simulink model "QuadCopterSimulation_CL_Original"  (R2024a)
settings: Solver=ode23t  StartTime=0  StopTime=25  RelTol=1e-6  AbsTol=1e-6
values from neighbouring files (symbols this model uses):
  Cd = 5.804e-9    (= 5.804e-09)    [parameters.m]
  Ct = 4.980e-8    (= 4.98e-08)    [parameters.m]
  d = 0.21    [parameters.m]
  g = 9.81    [parameters.m]
  Ixx = 1.467e-2    (= 0.01467)    [parameters.m]
  Iyy = 1.667e-2    (= 0.01667)    [parameters.m]
  Izz = 1.325e-2    (= 0.01325)    [parameters.m]
  m = 0.9    [parameters.m]
libraries: vrlib x9, slpidlib x4
settings Model: SimulationMode=accelerator  SnapshotInterval=1  PacingRate=1.300000  Creator=abdma  LastModifiedBy=abdma
settings SolverCC: AlgebraicLoopSolver=TrustRegion
settings DebuggingCC: UnconnectedInputMsg=warning  UnconnectedOutputMsg=warning  UnconnectedLineMsg=warning  ArithmeticOperatorsInVariantConditions=warning
settings ModelReferenceCC: EnableRefExpFcnMdlSchedulingChecks=on
settings SFSimCC: CustomCodeUndefinedFunction=UseInterfaceOnly
settings RTWCC: GPUComputeCapability=3.5

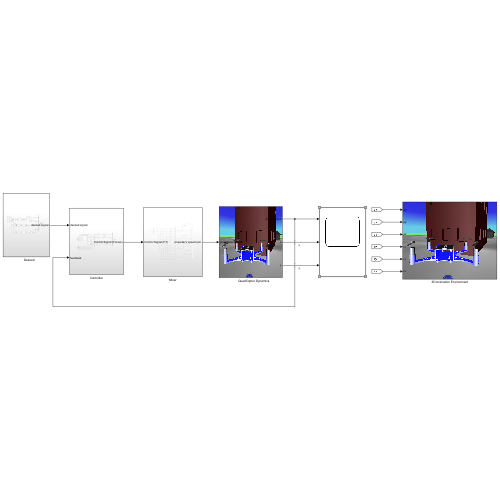
[thumbnail: Simulink's stored preview of the top-level diagram]
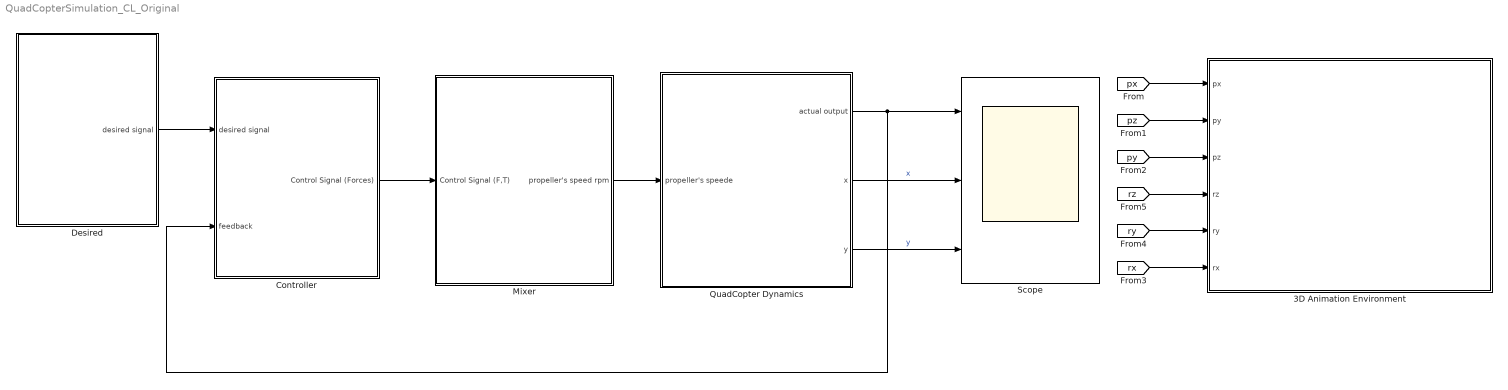
== system QuadCopterSimulation_CL_Original ==
  "\tDesired" : Subsystem
  "\tQuadCopter Dynamics" : Subsystem
      mask Display: image('Capture.PNG');
  3D Animation Environment : Subsystem
      mask Display: image('Capture.PNG');
  Controller : Subsystem
  Mixer : Subsystem
  Scope : Scope  NumInputPorts=3
  wires:
  "\tDesired"/1(desired signal) -> Controller/1(desired signal)
  Controller/1(Control Signal (Forces)) -> Mixer/1(Control Signal (F,T))
  "\tQuadCopter Dynamics"/1(actual output) -> Scope/1, Controller/2(feedback)
  Mixer/1(propeller's speed rpm) -> "\tQuadCopter Dynamics"/1(propeller's speede)
  "\tQuadCopter Dynamics"/2(x) -> Scope/2  "x"
  "\tQuadCopter Dynamics"/3(y) -> Scope/3  "y"
  [px] -> 3D Animation Environment/1(px)
  [pz] -> 3D Animation Environment/2(py)
  [py] -> 3D Animation Environment/3(pz)
  [rz] -> 3D Animation Environment/4(rz)
  [ry] -> 3D Animation Environment/5(ry)
  [rx] -> 3D Animation Environment/6(rx)

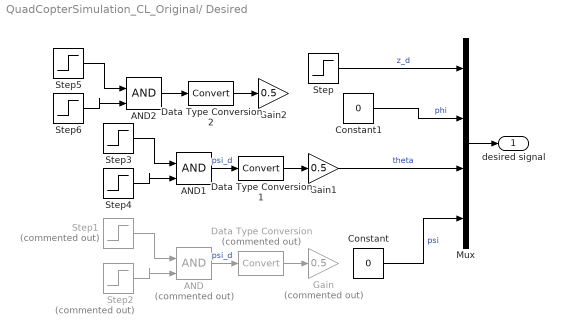
== system QuadCopterSimulation_CL_Original/	Desired ==
  AND : Logic  Commented=on  IconShape=distinctive  AllPortsSameDT=off  OutDataTypeStr=boolean
  AND1 : Logic  IconShape=distinctive  AllPortsSameDT=off  OutDataTypeStr=boolean
  AND2 : Logic  IconShape=distinctive  AllPortsSameDT=off  OutDataTypeStr=boolean
  Constant : Constant  Value=0
  Constant1 : Constant  Value=0
  Data Type Conversion : DataTypeConversion  Commented=on  SaturateOnIntegerOverflow=off  RndMeth=Floor
  Data Type Conversion1 : DataTypeConversion  SaturateOnIntegerOverflow=off  RndMeth=Floor
  Data Type Conversion2 : DataTypeConversion  SaturateOnIntegerOverflow=off  RndMeth=Floor
  Gain : Gain  Commented=on  Gain=0.5
  Gain1 : Gain  Gain=0.5
  Gain2 : Gain  Gain=0.5
  Mux : Mux
  Step : Step  Time=0  After=-5  SampleTime=0
  Step1 : Step  Commented=on  Time=4  SampleTime=0
  Step2 : Step  Commented=on  Time=8  Before=1  After=0  SampleTime=0
  Step3 : Step  Time=8  SampleTime=0
  Step4 : Step  Time=9  Before=1  After=0  SampleTime=0
  Step5 : Step  Time=10  SampleTime=0
  Step6 : Step  Time=11  Before=1  After=0  SampleTime=0
  desired signal : Outport
  wires:
  Step/1 -> Mux/1  "z_d"
  AND/1 -> Data Type Conversion/1  "psi_d"
  Mux/1 -> desired signal/1
  Step1/1 -> AND/1
  Step2/1 -> AND/2
  Data Type Conversion/1 -> Gain/1
  Data Type Conversion1/1 -> Gain1/1
  Step4/1 -> AND1/2
  Step3/1 -> AND1/1
  AND1/1 -> Data Type Conversion1/1  "psi_d"
  Constant/1 -> Mux/4  "psi"
  Gain1/1 -> Mux/3  "theta"
  AND2/1 -> Data Type Conversion2/1
  Step5/1 -> AND2/1
  Step6/1 -> AND2/2
  Data Type Conversion2/1 -> Gain2/1
  Constant1/1 -> Mux/2  "phi"

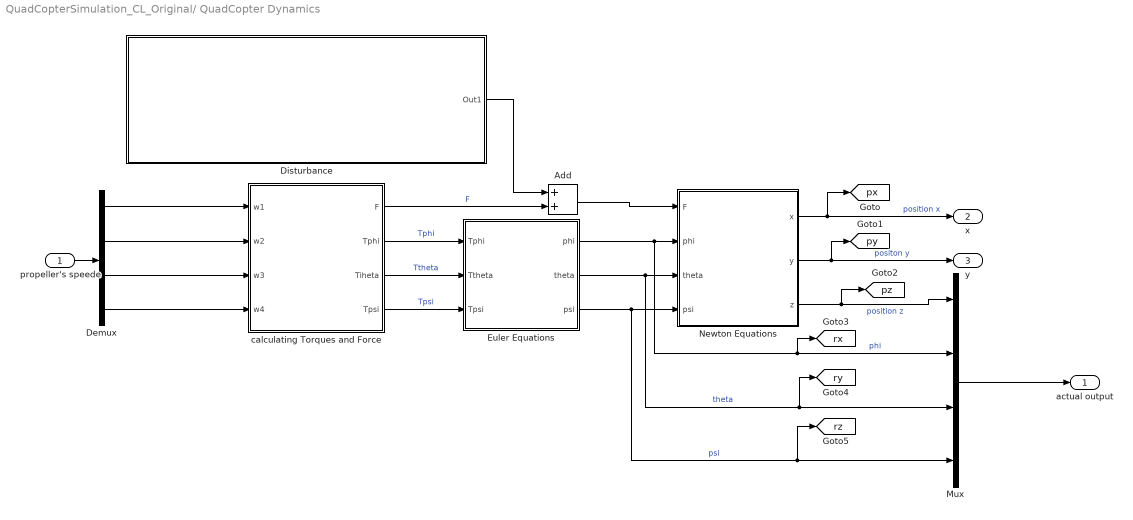
== system QuadCopterSimulation_CL_Original/	QuadCopter Dynamics ==
  propeller's speede : Inport
  Add : Sum
  Demux : Demux
  Disturbance : Subsystem
  Euler Equations : Subsystem
  Mux : Mux
  Newton Equations : Subsystem
  calculating Torques and Force : Subsystem
  actual output : Outport
  x : Outport  Port=2
  y : Outport  Port=3
  tag scope: px=global, py=global, pz=global, rx=global, ry=global, rz=global
  wires:
  Euler Equations/1(phi) -> [rx], Mux/2, Newton Equations/2(phi)  "phi"
  Euler Equations/3(psi) -> [rz], Mux/4, Newton Equations/4(psi)  "psi"
  calculating Torques and Force/3(Tiheta) -> Euler Equations/2(Ttheta)  "Ttheta"
  Euler Equations/2(theta) -> [ry], Mux/3, Newton Equations/3(theta)  "theta"
  calculating Torques and Force/2(Tphi) -> Euler Equations/1(Tphi)  "Tphi"
  Newton Equations/1(x) -> [px], x/1  "position x"
  calculating Torques and Force/4(Tpsi) -> Euler Equations/3(Tpsi)  "Tpsi"
  Newton Equations/2(y) -> [py], y/1  "positon y"
  Newton Equations/3(z) -> [pz], Mux/1  "position z"
  Mux/1 -> actual output/1
  propeller's speede/1 -> Demux/1
  Demux/1 -> calculating Torques and Force/1(w1)
  Demux/2 -> calculating Torques and Force/2(w2)
  Demux/3 -> calculating Torques and Force/3(w3)
  Demux/4 -> calculating Torques and Force/4(w4)
  calculating Torques and Force/1(F) -> Add/2  "F"
  Add/1 -> Newton Equations/1(F)
  Disturbance/1(Out1) -> Add/1

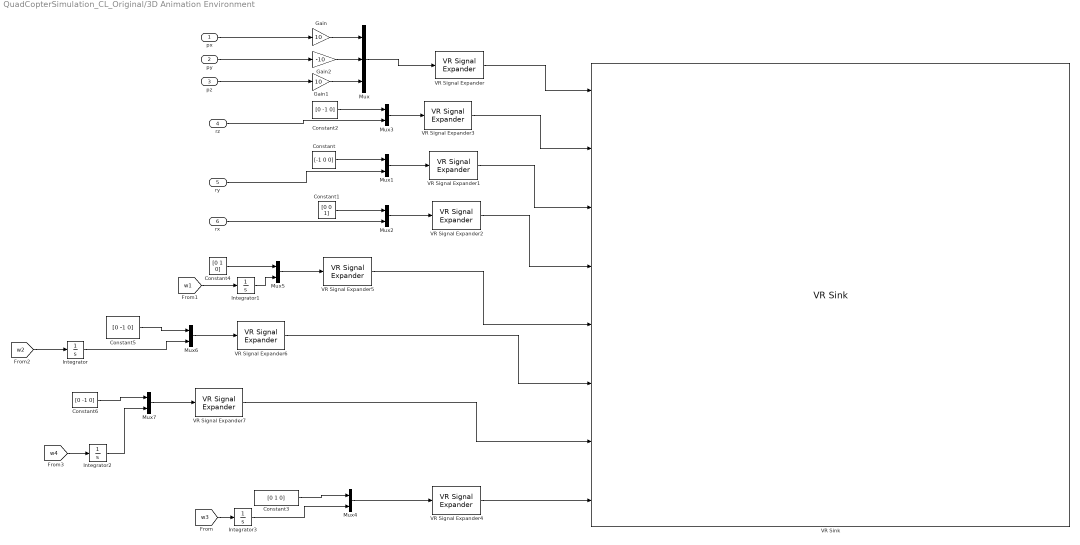
== system QuadCopterSimulation_CL_Original/3D Animation Environment ==
  px : Inport
  py : Inport  Port=2
  pz : Inport  Port=3
  rz : Inport  Port=4
  ry : Inport  Port=5
  rx : Inport  Port=6
  Constant : Constant  Value=[-1 0 0]
  Constant1 : Constant  Value=[0 0 1]
  Constant2 : Constant  Value=[0 -1 0]
  Constant3 : Constant  Value=[0 1 0]
  Constant4 : Constant  Value=[0 1 0]
  Constant5 : Constant  Value=[0 -1 0]
  Constant6 : Constant  Value=[0 -1 0]
  Gain : Gain  Gain=10
  Gain1 : Gain  Gain=10
  Gain2 : Gain  Gain=-10
  Integrator{,1..3} (4 alike) : Integrator
  Mux : Mux  Inputs=3
  Mux{1..7} (7 alike) : Mux  Inputs=2
  VR Signal Expander : vrlib/VR Signal Expander  outwidth=3  outidx=[1 2 3 ]
  VR Signal Expander{1..7} (7 alike) : vrlib/VR Signal Expander  outwidth=4  outidx=[1 2 3 4]
  VR Sink : vrlib/VR Sink  InstantiateOnLoad=on  SampleTime=0.1  ViewEnable=on  RemoteChange=off  RemoteView=off  FieldsWritten=DroneFrame.translation.3.1.1.double#frameZ.rotation.4.1.1.double#frameY.rotation.4.1.1.double#frameX.rotation.4.1.1.double#propeller1.rotation.4.1.1.double#propeller2.rotation.4.1.1.double#propeller4.rotation.4.1.1.double#propeller3.rotation.4.1.1.double  WorldFileName=minidroneassembly.wrl  AutoView=on  VideoDimensions=[]  AllowVariableSize=off
  wires:
  Mux/1 -> VR Signal Expander/1
  Mux3/1 -> VR Signal Expander3/1
  Gain2/1 -> Mux/2
  Gain1/1 -> Mux/3
  rx/1 -> Mux2/2
  Mux1/1 -> VR Signal Expander1/1
  Gain/1 -> Mux/1
  rz/1 -> Mux3/2
  Constant/1 -> Mux1/1
  Mux2/1 -> VR Signal Expander2/1
  Constant2/1 -> Mux3/1
  Constant1/1 -> Mux2/1
  ry/1 -> Mux1/2
  pz/1 -> Gain1/1
  px/1 -> Gain/1
  py/1 -> Gain2/1
  Constant3/1 -> Mux4/1
  Mux4/1 -> VR Signal Expander4/1
  [w3] -> Integrator3/1
  VR Signal Expander/1 -> VR Sink/1
  VR Signal Expander3/1 -> VR Sink/2
  VR Signal Expander1/1 -> VR Sink/3
  VR Signal Expander2/1 -> VR Sink/4
  VR Signal Expander4/1 -> VR Sink/8
  VR Signal Expander5/1 -> VR Sink/5
  [w1] -> Integrator1/1
  Mux5/1 -> VR Signal Expander5/1
  Constant4/1 -> Mux5/1
  Constant5/1 -> Mux6/1
  Mux6/1 -> VR Signal Expander6/1
  [w2] -> Integrator/1
  VR Signal Expander6/1 -> VR Sink/6
  VR Signal Expander7/1 -> VR Sink/7
  [w4] -> Integrator2/1
  Mux7/1 -> VR Signal Expander7/1
  Constant6/1 -> Mux7/1
  Integrator/1 -> Mux6/2
  Integrator1/1 -> Mux5/2
  Integrator2/1 -> Mux7/2
  Integrator3/1 -> Mux4/2

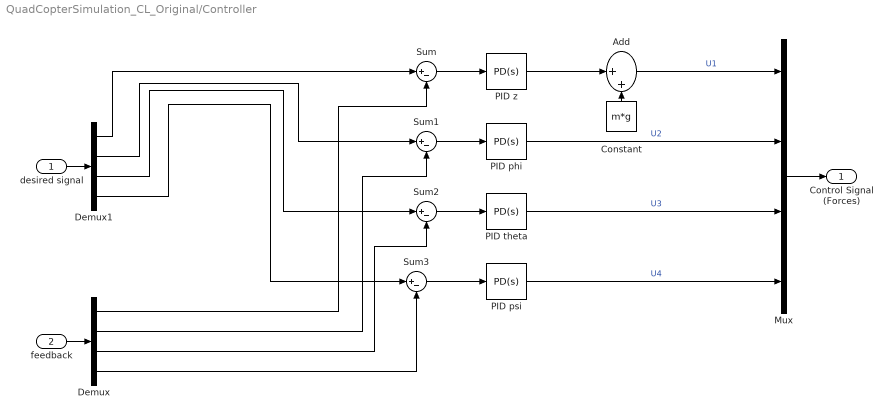
== system QuadCopterSimulation_CL_Original/Controller ==
  desired signal : Inport
  feedback : Inport  Port=2
  Add : Sum  Inputs=|++
  Constant : Constant  Value=m*g
  Demux : Demux
  Demux1 : Demux
  Mux : Mux
  PID phi : slpidlib/PID Controller  Controller=PD  Form=Parallel  TimeDomain=Continuous-time  UseExternalTs=off  SampleTime=-1  IntegratorMethod=Forward Euler  FilterMethod=Forward Euler  ControllerParametersSource=internal  P=3.08e-3  I=1  UseKiTs=off  D=1.43e-2  UseExternalDerivativeSource=off  N=114.286  UseFilter=on  TunerSelectOption=Transfer Function Based (PID Tuner App)  InitialConditionSource=internal  InitialConditionForIntegrator=0  InitialConditionForFilter=0  DifferentiatorICPrevScaledInput=0  ExternalReset=none  TrackingMode=off  Kt=1  LimitOutput=off  SatLimitsSource=internal  UpperSaturationLimit=inf  LowerSaturationLimit=-inf  LinearizeAsGain=on  AntiWindupMode=none  Kb=1  LimitIntegrator=off  UpperIntegratorSaturationLimit=inf  LowerIntegratorSaturationLimit=-inf  POutMin=[]  POutMax=[]  IOutMin=[]  IOutMax=[]  DOutMin=[]  DOutMax=[]  NOutMin=[]  NOutMax=[]  SumOutMin=[]  SumOutMax=[]  SaturationOutMin=[]  SaturationOutMax=[]  PParamMin=[]  PParamMax=[]  IParamMin=[]  IParamMax=[]  DParamMin=[]  DParamMax=[]  NParamMin=[]  NParamMax=[]  KbParamMin=[]  KbParamMax=[]  KtParamMin=[]  KtParamMax=[]  KbOutMin=[]  KbOutMax=[]  KtOutMin=[]  KtOutMax=[]  IntegratorOutMin=[]  IntegratorOutMax=[]  FilterOutMin=[]  FilterOutMax=[]  SumI1OutMin=[]  SumI1OutMax=[]  SumI2OutMin=[]  SumI2OutMax=[]  SumI3OutMin=[]  SumI3OutMax=[]  SumI4OutMin=[]  SumI4OutMax=[]  SumDOutMin=[]  SumDOutMax=[]  DifferentiatorOutMin=[]  DifferentiatorOutMax=[]  FilterDiffOutCoefMin=[]  FilterDiffOutCoefMax=[]  ReciprocalOutMin=[]  ReciprocalOutMax=[]  SumDenOutMin=[]  SumDenOutMax=[]  SumNumOutMin=[]  SumNumOutMax=[]  DivideOutMin=[]  DivideOutMax=[]  UdiffTsProdOutMin=[]  UdiffTsProdOutMax=[]  NTsProdOutMin=[]  NTsProdOutMax=[]  UintegralTsProdOutMin=[]  UintegralTsProdOutMax=[]  UngainTsProdOutMin=[]  UngainTsProdOutMax=[]  ClampingZeroOutDataTypeStr=Inherit: Inherit via back propagation  ClampingZeroOutMin=[]  ClampingZeroOutMax=[]  FilterDenConstantOutDataTypeStr=Inherit: Inherit via back propagation  FilterDenConstantOutMin=[]  FilterDenConstantOutMax=[]  PCopyOutDataTypeStr=Inherit: Inherit via back propagation  PCopyOutMin=[]  PCopyOutMax=[]  NCopyOutDataTypeStr=Inherit: Inherit via back propagation  NCopyOutMin=[]  NCopyOutMax=[]  IntegratorContinuousStateAttributes=''  IntegratorStateMustResolveToSignalObject=off  IntegratorRTWStateStorageClass=Auto  FilterContinuousStateAttributes=''  FilterStateMustResolveToSignalObject=off  FilterRTWStateStorageClass=Auto  ParallelPVariant=InternalParameters  IdealPVariant=Disabled  IVariant=Disabled  DVariant=InternalParameters  IntegratorVariant=Disabled  SatVariant=Disabled  AWVariant=Disabled  PCopyVariant=Disabled  TRVariant=Disabled  FdbkBlocksVariant=Forward  IdealPFdbkVariant=Disabled  SatFdbkVariant=Disabled  DerivativeFilterVariant=ContFilter  NVariant=InternalParameters  NCopyVariant=Disabled  FilterICVariant=InternalICsFilter  IntegratorICVariant=Disabled  ExternalResetVariant=Disabled  TRSumVariant=Passthrough  SumFdbkVariant=Disabled  SumVariant=Sum_PD  TsampFilterVariant=InternalTs  TsampNgainVariant=Passthrough  TsampIntegralVariant=Disabled_SignalSpec  ExternalSaturationOutDataTypeStr=Inherit: Same as second input  DerivativeSourceVariant=ErrorSignal
  PID psi : slpidlib/PID Controller  Controller=PD  Form=Parallel  TimeDomain=Continuous-time  UseExternalTs=off  SampleTime=-1  IntegratorMethod=Forward Euler  FilterMethod=Forward Euler  ControllerParametersSource=internal  P=3.08e-3  I=1  UseKiTs=off  D=1.43e-2  UseExternalDerivativeSource=off  N=114.286  UseFilter=on  TunerSelectOption=Transfer Function Based (PID Tuner App)  InitialConditionSource=internal  InitialConditionForIntegrator=0  InitialConditionForFilter=0  DifferentiatorICPrevScaledInput=0  ExternalReset=none  TrackingMode=off  Kt=1  LimitOutput=off  SatLimitsSource=internal  UpperSaturationLimit=inf  LowerSaturationLimit=-inf  LinearizeAsGain=on  AntiWindupMode=none  Kb=1  LimitIntegrator=off  UpperIntegratorSaturationLimit=inf  LowerIntegratorSaturationLimit=-inf  POutMin=[]  POutMax=[]  IOutMin=[]  IOutMax=[]  DOutMin=[]  DOutMax=[]  NOutMin=[]  NOutMax=[]  SumOutMin=[]  SumOutMax=[]  SaturationOutMin=[]  SaturationOutMax=[]  PParamMin=[]  PParamMax=[]  IParamMin=[]  IParamMax=[]  DParamMin=[]  DParamMax=[]  NParamMin=[]  NParamMax=[]  KbParamMin=[]  KbParamMax=[]  KtParamMin=[]  KtParamMax=[]  KbOutMin=[]  KbOutMax=[]  KtOutMin=[]  KtOutMax=[]  IntegratorOutMin=[]  IntegratorOutMax=[]  FilterOutMin=[]  FilterOutMax=[]  SumI1OutMin=[]  SumI1OutMax=[]  SumI2OutMin=[]  SumI2OutMax=[]  SumI3OutMin=[]  SumI3OutMax=[]  SumI4OutMin=[]  SumI4OutMax=[]  SumDOutMin=[]  SumDOutMax=[]  DifferentiatorOutMin=[]  DifferentiatorOutMax=[]  FilterDiffOutCoefMin=[]  FilterDiffOutCoefMax=[]  ReciprocalOutMin=[]  ReciprocalOutMax=[]  SumDenOutMin=[]  SumDenOutMax=[]  SumNumOutMin=[]  SumNumOutMax=[]  DivideOutMin=[]  DivideOutMax=[]  UdiffTsProdOutMin=[]  UdiffTsProdOutMax=[]  NTsProdOutMin=[]  NTsProdOutMax=[]  UintegralTsProdOutMin=[]  UintegralTsProdOutMax=[]  UngainTsProdOutMin=[]  UngainTsProdOutMax=[]  ClampingZeroOutDataTypeStr=Inherit: Inherit via back propagation  ClampingZeroOutMin=[]  ClampingZeroOutMax=[]  FilterDenConstantOutDataTypeStr=Inherit: Inherit via back propagation  FilterDenConstantOutMin=[]  FilterDenConstantOutMax=[]  PCopyOutDataTypeStr=Inherit: Inherit via back propagation  PCopyOutMin=[]  PCopyOutMax=[]  NCopyOutDataTypeStr=Inherit: Inherit via back propagation  NCopyOutMin=[]  NCopyOutMax=[]  IntegratorContinuousStateAttributes=''  IntegratorStateMustResolveToSignalObject=off  IntegratorRTWStateStorageClass=Auto  FilterContinuousStateAttributes=''  FilterStateMustResolveToSignalObject=off  FilterRTWStateStorageClass=Auto  ParallelPVariant=InternalParameters  IdealPVariant=Disabled  IVariant=Disabled  DVariant=InternalParameters  IntegratorVariant=Disabled  SatVariant=Disabled  AWVariant=Disabled  PCopyVariant=Disabled  TRVariant=Disabled  FdbkBlocksVariant=Forward  IdealPFdbkVariant=Disabled  SatFdbkVariant=Disabled  DerivativeFilterVariant=ContFilter  NVariant=InternalParameters  NCopyVariant=Disabled  FilterICVariant=InternalICsFilter  IntegratorICVariant=Disabled  ExternalResetVariant=Disabled  TRSumVariant=Passthrough  SumFdbkVariant=Disabled  SumVariant=Sum_PD  TsampFilterVariant=InternalTs  TsampNgainVariant=Passthrough  TsampIntegralVariant=Disabled_SignalSpec  ExternalSaturationOutDataTypeStr=Inherit: Same as second input  DerivativeSourceVariant=ErrorSignal
  PID theta : slpidlib/PID Controller  Controller=PD  Form=Parallel  TimeDomain=Continuous-time  UseExternalTs=off  SampleTime=-1  IntegratorMethod=Forward Euler  FilterMethod=Forward Euler  ControllerParametersSource=internal  P=3.08e-3  I=1  UseKiTs=off  D=1.43e-2  UseExternalDerivativeSource=off  N=114.286  UseFilter=on  TunerSelectOption=Transfer Function Based (PID Tuner App)  InitialConditionSource=internal  InitialConditionForIntegrator=0  InitialConditionForFilter=0  DifferentiatorICPrevScaledInput=0  ExternalReset=none  TrackingMode=off  Kt=1  LimitOutput=off  SatLimitsSource=internal  UpperSaturationLimit=inf  LowerSaturationLimit=-inf  LinearizeAsGain=on  AntiWindupMode=none  Kb=1  LimitIntegrator=off  UpperIntegratorSaturationLimit=inf  LowerIntegratorSaturationLimit=-inf  POutMin=[]  POutMax=[]  IOutMin=[]  IOutMax=[]  DOutMin=[]  DOutMax=[]  NOutMin=[]  NOutMax=[]  SumOutMin=[]  SumOutMax=[]  SaturationOutMin=[]  SaturationOutMax=[]  PParamMin=[]  PParamMax=[]  IParamMin=[]  IParamMax=[]  DParamMin=[]  DParamMax=[]  NParamMin=[]  NParamMax=[]  KbParamMin=[]  KbParamMax=[]  KtParamMin=[]  KtParamMax=[]  KbOutMin=[]  KbOutMax=[]  KtOutMin=[]  KtOutMax=[]  IntegratorOutMin=[]  IntegratorOutMax=[]  FilterOutMin=[]  FilterOutMax=[]  SumI1OutMin=[]  SumI1OutMax=[]  SumI2OutMin=[]  SumI2OutMax=[]  SumI3OutMin=[]  SumI3OutMax=[]  SumI4OutMin=[]  SumI4OutMax=[]  SumDOutMin=[]  SumDOutMax=[]  DifferentiatorOutMin=[]  DifferentiatorOutMax=[]  FilterDiffOutCoefMin=[]  FilterDiffOutCoefMax=[]  ReciprocalOutMin=[]  ReciprocalOutMax=[]  SumDenOutMin=[]  SumDenOutMax=[]  SumNumOutMin=[]  SumNumOutMax=[]  DivideOutMin=[]  DivideOutMax=[]  UdiffTsProdOutMin=[]  UdiffTsProdOutMax=[]  NTsProdOutMin=[]  NTsProdOutMax=[]  UintegralTsProdOutMin=[]  UintegralTsProdOutMax=[]  UngainTsProdOutMin=[]  UngainTsProdOutMax=[]  ClampingZeroOutDataTypeStr=Inherit: Inherit via back propagation  ClampingZeroOutMin=[]  ClampingZeroOutMax=[]  FilterDenConstantOutDataTypeStr=Inherit: Inherit via back propagation  FilterDenConstantOutMin=[]  FilterDenConstantOutMax=[]  PCopyOutDataTypeStr=Inherit: Inherit via back propagation  PCopyOutMin=[]  PCopyOutMax=[]  NCopyOutDataTypeStr=Inherit: Inherit via back propagation  NCopyOutMin=[]  NCopyOutMax=[]  IntegratorContinuousStateAttributes=''  IntegratorStateMustResolveToSignalObject=off  IntegratorRTWStateStorageClass=Auto  FilterContinuousStateAttributes=''  FilterStateMustResolveToSignalObject=off  FilterRTWStateStorageClass=Auto  ParallelPVariant=InternalParameters  IdealPVariant=Disabled  IVariant=Disabled  DVariant=InternalParameters  IntegratorVariant=Disabled  SatVariant=Disabled  AWVariant=Disabled  PCopyVariant=Disabled  TRVariant=Disabled  FdbkBlocksVariant=Forward  IdealPFdbkVariant=Disabled  SatFdbkVariant=Disabled  DerivativeFilterVariant=ContFilter  NVariant=InternalParameters  NCopyVariant=Disabled  FilterICVariant=InternalICsFilter  IntegratorICVariant=Disabled  ExternalResetVariant=Disabled  TRSumVariant=Passthrough  SumFdbkVariant=Disabled  SumVariant=Sum_PD  TsampFilterVariant=InternalTs  TsampNgainVariant=Passthrough  TsampIntegralVariant=Disabled_SignalSpec  ExternalSaturationOutDataTypeStr=Inherit: Same as second input  DerivativeSourceVariant=ErrorSignal
  PID z : slpidlib/PID Controller  Controller=PD  Form=Parallel  TimeDomain=Continuous-time  UseExternalTs=off  SampleTime=-1  IntegratorMethod=Forward Euler  FilterMethod=Forward Euler  ControllerParametersSource=internal  P=100e-2  I=1  UseKiTs=off  D=100e-2  UseExternalDerivativeSource=off  N=114.286  UseFilter=on  TunerSelectOption=Transfer Function Based (PID Tuner App)  InitialConditionSource=internal  InitialConditionForIntegrator=0  InitialConditionForFilter=0  DifferentiatorICPrevScaledInput=0  ExternalReset=none  TrackingMode=off  Kt=1  LimitOutput=off  SatLimitsSource=internal  UpperSaturationLimit=inf  LowerSaturationLimit=-inf  LinearizeAsGain=on  AntiWindupMode=none  Kb=1  LimitIntegrator=off  UpperIntegratorSaturationLimit=inf  LowerIntegratorSaturationLimit=-inf  POutMin=[]  POutMax=[]  IOutMin=[]  IOutMax=[]  DOutMin=[]  DOutMax=[]  NOutMin=[]  NOutMax=[]  SumOutMin=[]  SumOutMax=[]  SaturationOutMin=[]  SaturationOutMax=[]  PParamMin=[]  PParamMax=[]  IParamMin=[]  IParamMax=[]  DParamMin=[]  DParamMax=[]  NParamMin=[]  NParamMax=[]  KbParamMin=[]  KbParamMax=[]  KtParamMin=[]  KtParamMax=[]  KbOutMin=[]  KbOutMax=[]  KtOutMin=[]  KtOutMax=[]  IntegratorOutMin=[]  IntegratorOutMax=[]  FilterOutMin=[]  FilterOutMax=[]  SumI1OutMin=[]  SumI1OutMax=[]  SumI2OutMin=[]  SumI2OutMax=[]  SumI3OutMin=[]  SumI3OutMax=[]  SumI4OutMin=[]  SumI4OutMax=[]  SumDOutMin=[]  SumDOutMax=[]  DifferentiatorOutMin=[]  DifferentiatorOutMax=[]  FilterDiffOutCoefMin=[]  FilterDiffOutCoefMax=[]  ReciprocalOutMin=[]  ReciprocalOutMax=[]  SumDenOutMin=[]  SumDenOutMax=[]  SumNumOutMin=[]  SumNumOutMax=[]  DivideOutMin=[]  DivideOutMax=[]  UdiffTsProdOutMin=[]  UdiffTsProdOutMax=[]  NTsProdOutMin=[]  NTsProdOutMax=[]  UintegralTsProdOutMin=[]  UintegralTsProdOutMax=[]  UngainTsProdOutMin=[]  UngainTsProdOutMax=[]  ClampingZeroOutDataTypeStr=Inherit: Inherit via back propagation  ClampingZeroOutMin=[]  ClampingZeroOutMax=[]  FilterDenConstantOutDataTypeStr=Inherit: Inherit via back propagation  FilterDenConstantOutMin=[]  FilterDenConstantOutMax=[]  PCopyOutDataTypeStr=Inherit: Inherit via back propagation  PCopyOutMin=[]  PCopyOutMax=[]  NCopyOutDataTypeStr=Inherit: Inherit via back propagation  NCopyOutMin=[]  NCopyOutMax=[]  IntegratorContinuousStateAttributes=''  IntegratorStateMustResolveToSignalObject=off  IntegratorRTWStateStorageClass=Auto  FilterContinuousStateAttributes=''  FilterStateMustResolveToSignalObject=off  FilterRTWStateStorageClass=Auto  ParallelPVariant=InternalParameters  IdealPVariant=Disabled  IVariant=Disabled  DVariant=InternalParameters  IntegratorVariant=Disabled  SatVariant=Disabled  AWVariant=Disabled  PCopyVariant=Disabled  TRVariant=Disabled  FdbkBlocksVariant=Forward  IdealPFdbkVariant=Disabled  SatFdbkVariant=Disabled  DerivativeFilterVariant=ContFilter  NVariant=InternalParameters  NCopyVariant=Disabled  FilterICVariant=InternalICsFilter  IntegratorICVariant=Disabled  ExternalResetVariant=Disabled  TRSumVariant=Passthrough  SumFdbkVariant=Disabled  SumVariant=Sum_PD  TsampFilterVariant=InternalTs  TsampNgainVariant=Passthrough  TsampIntegralVariant=Disabled_SignalSpec  ExternalSaturationOutDataTypeStr=Inherit: Same as second input  DerivativeSourceVariant=ErrorSignal
  Sum{,1..3} (4 alike) : Sum  Inputs=|+-
  Control Signal (Forces) : Outport
  wires:
  Demux/4 -> Sum3/2
  Sum/1 -> PID z/1
  Demux/3 -> Sum2/2
  Demux1/4 -> Sum3/1
  Sum3/1 -> PID psi/1
  Sum2/1 -> PID theta/1
  Sum1/1 -> PID phi/1
  Demux1/1 -> Sum/1
  PID phi/1 -> Mux/2  "U2"
  PID theta/1 -> Mux/3  "U3"
  Demux1/2 -> Sum1/1
  Demux/2 -> Sum1/2
  Demux1/3 -> Sum2/1
  PID psi/1 -> Mux/4  "U4"
  Demux/1 -> Sum/2
  PID z/1 -> Add/1
  Add/1 -> Mux/1  "U1"
  Constant/1 -> Add/2
  feedback/1 -> Demux/1
  desired signal/1 -> Demux1/1
  Mux/1 -> Control Signal (Forces)/1

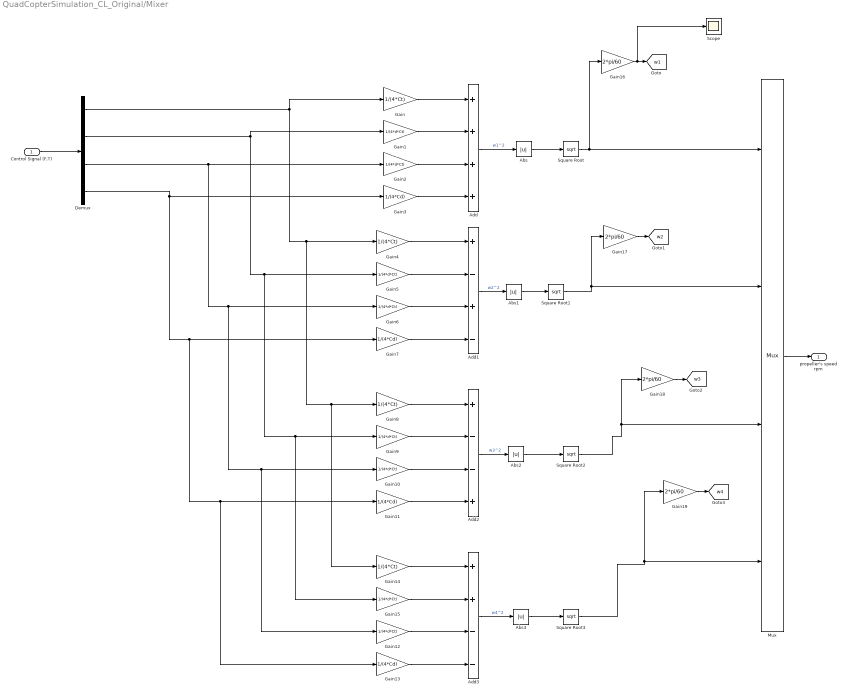
== system QuadCopterSimulation_CL_Original/Mixer ==
  Control Signal (F,T) : Inport
  Abs{,1..3} (4 alike) : Abs  SaturateOnIntegerOverflow=off
  Add : Sum  Inputs=++++
  Add1 : Sum  Inputs=+-+-
  Add2 : Sum  Inputs=+--+
  Add3 : Sum  Inputs=++--
  Demux : Demux
  Gain{,4,8,14} (4 alike) : Gain  Gain=1/(4*Ct)
  Gain{1..2,5..6,9..10,12,15} (8 alike) : Gain  Gain=1/(4*d*Ct)
  Gain{3,7,11,13} (4 alike) : Gain  Gain=1/(4*Cd)
  Gain{16..19} (4 alike) : Gain  Gain=2*pi/60
  Mux : Mux
  Scope : Scope
  Square Root{,1..3} (4 alike) : Sqrt
  propeller's speed rpm : Outport
  tag scope: w1=global, w2=global, w3=global, w4=global
  wires:
  Gain/1 -> Add/1
  Demux/3 -> Gain12/1, Gain10/1, Gain6/1, Gain2/1
  Gain3/1 -> Add/4
  Gain1/1 -> Add/2
  Demux/2 -> Gain1/1, Gain15/1, Gain9/1, Gain5/1
  Gain2/1 -> Add/3
  Add/1 -> Abs/1  "w1^2"
  Add1/1 -> Abs1/1  "w2^2"
  Gain6/1 -> Add1/3
  Gain5/1 -> Add1/2
  Gain7/1 -> Add1/4
  Demux/1 -> Gain/1, Gain4/1, Gain14/1, Gain8/1
  Gain4/1 -> Add1/1
  Gain8/1 -> Add2/1
  Gain11/1 -> Add2/4
  Gain9/1 -> Add2/2
  Gain10/1 -> Add2/3
  Add2/1 -> Abs2/1  "w3^2"
  Gain13/1 -> Add3/4
  Gain12/1 -> Add3/3
  Add3/1 -> Abs3/1  "w4^2"
  Gain14/1 -> Add3/1
  Gain15/1 -> Add3/2
  Demux/4 -> Gain13/1, Gain11/1, Gain7/1, Gain3/1
  Abs/1 -> Square Root/1
  Abs1/1 -> Square Root1/1
  Abs2/1 -> Square Root2/1
  Abs3/1 -> Square Root3/1
  Control Signal (F,T)/1 -> Demux/1
  Mux/1 -> propeller's speed rpm/1
  Square Root/1 -> Gain16/1, Mux/1
  Gain16/1 -> Scope/1, [w1]
  Gain17/1 -> [w2]
  Square Root1/1 -> Gain17/1, Mux/2
  Square Root2/1 -> Gain18/1, Mux/3
  Gain18/1 -> [w3]
  Gain19/1 -> [w4]
  Square Root3/1 -> Gain19/1, Mux/4

== system QuadCopterSimulation_CL_Original/	QuadCopter Dynamics/Disturbance ==
  AND : Logic  IconShape=distinctive  AllPortsSameDT=off  OutDataTypeStr=boolean
  Data Type Conversion : DataTypeConversion  SaturateOnIntegerOverflow=off  RndMeth=Floor
  Gain : Gain  Gain=5
  Step : Step  Time=10  SampleTime=0
  Step1 : Step  Time=11  Before=1  After=0  SampleTime=0
  Out1 : Outport
  wires:
  Step/1 -> AND/1
  AND/1 -> Data Type Conversion/1
  Step1/1 -> AND/2
  Data Type Conversion/1 -> Gain/1
  Gain/1 -> Out1/1

== system QuadCopterSimulation_CL_Original/	QuadCopter Dynamics/Euler Equations ==
  Tphi : Inport
  Ttheta : Inport  Port=2
  Tpsi : Inport  Port=3
  Subsystem : Subsystem
  Subsystem1 : Subsystem
  Subsystem2 : Subsystem
  p_q _r_equations : Subsystem
  phi : Outport
  theta : Outport  Port=2
  psi : Outport  Port=3
  wires:
  p_q _r_equations/3(r) -> Subsystem2/2(r), Subsystem/3(r), Subsystem1/2(r)
  Subsystem/1(phi) -> phi/1, Subsystem2/3(phi), Subsystem1/1(phi)  "phi"
  Subsystem1/1(theta) -> Subsystem2/4(theta), Subsystem/4(theta), theta/1  "theta"
  Tphi/1 -> p_q _r_equations/1(Tphi)
  p_q _r_equations/2(q) -> Subsystem1/3(q), Subsystem2/1(q), Subsystem/2(q)
  p_q _r_equations/1(p) -> Subsystem/1(p)
  Subsystem2/1(psi) -> psi/1
  Ttheta/1 -> p_q _r_equations/2(Ttheta)
  Tpsi/1 -> p_q _r_equations/3(Tpsi)

== system QuadCopterSimulation_CL_Original/	QuadCopter Dynamics/Newton Equations ==
  F : Inport
  phi : Inport  Port=2
  theta : Inport  Port=3
  psi : Inport  Port=4
  Subsystem : Subsystem
  Subsystem1 : Subsystem
  Subsystem2 : Subsystem
  x : Outport
  y : Outport  Port=2
  z : Outport  Port=3
  wires:
  Subsystem/1(x) -> x/1
  theta/1 -> Subsystem/3(theta), Subsystem2/3(theta), Subsystem1/3(theta)
  F/1 -> Subsystem2/1(F), Subsystem1/1(F), Subsystem/1(F)
  phi/1 -> Subsystem/2(phi), Subsystem2/2(phi), Subsystem1/2(phi)
  Subsystem2/1(z) -> z/1
  Subsystem1/1(y) -> y/1
  psi/1 -> Subsystem/4(psi), Subsystem1/4(psi)

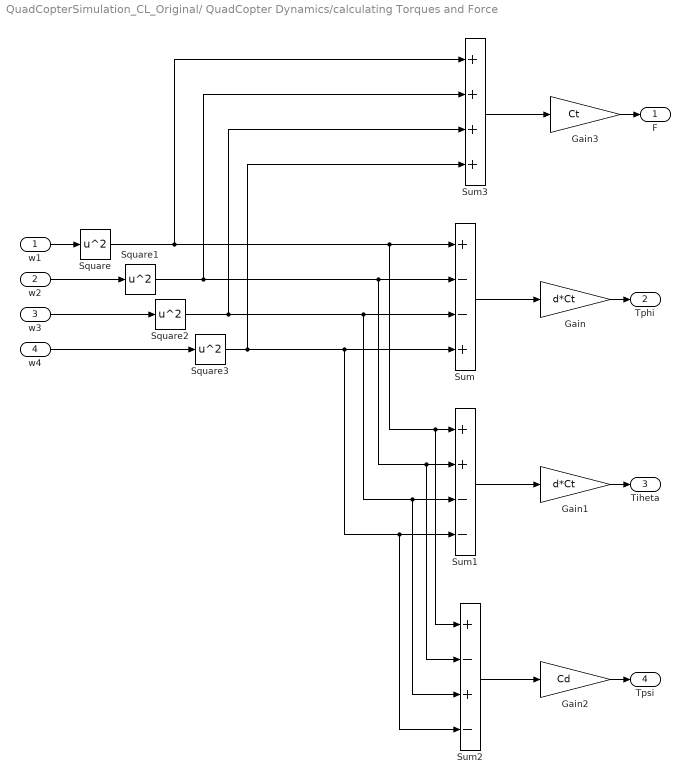
== system QuadCopterSimulation_CL_Original/	QuadCopter Dynamics/calculating Torques and Force ==
  w1 : Inport
  w2 : Inport  Port=2
  w3 : Inport  Port=3
  w4 : Inport  Port=4
  Gain : Gain  Gain=d*Ct
  Gain1 : Gain  Gain=d*Ct
  Gain2 : Gain  Gain=Cd
  Gain3 : Gain  Gain=Ct
  Square{,1..3} (4 alike) : Math  Operator=square  SignedPower=on
  Sum : Sum  Inputs=+--+
  Sum1 : Sum  Inputs=++--
  Sum2 : Sum  Inputs=+-+-
  Sum3 : Sum  Inputs=++++
  F : Outport
  Tphi : Outport  Port=2
  Tiheta : Outport  Port=3
  Tpsi : Outport  Port=4
  wires:
  w2/1 -> Square1/1
  w1/1 -> Square/1
  w3/1 -> Square2/1
  w4/1 -> Square3/1
  Sum/1 -> Gain/1
  Sum3/1 -> Gain3/1
  Gain3/1 -> F/1
  Gain1/1 -> Tiheta/1
  Sum2/1 -> Gain2/1
  Sum1/1 -> Gain1/1
  Gain2/1 -> Tpsi/1
  Gain/1 -> Tphi/1
  Square/1 -> Sum3/1, Sum2/1, Sum1/1, Sum/1
  Square1/1 -> Sum3/2, Sum2/2, Sum1/2, Sum/2
  Square2/1 -> Sum3/3, Sum2/3, Sum1/3, Sum/3
  Square3/1 -> Sum3/4, Sum2/4, Sum1/4, Sum/4

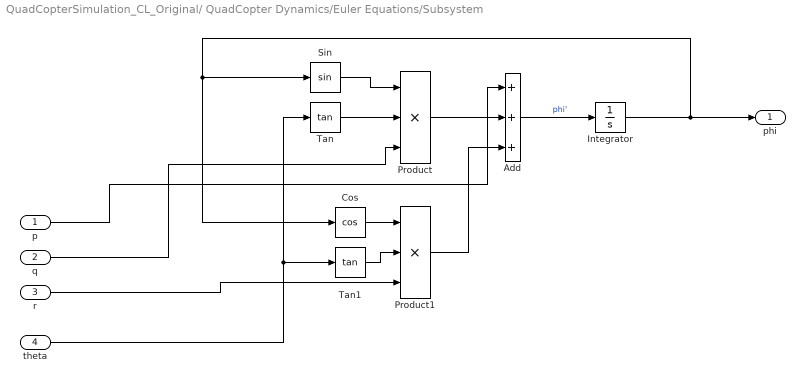
== system QuadCopterSimulation_CL_Original/	QuadCopter Dynamics/Euler Equations/Subsystem ==
  p : Inport
  q : Inport  Port=2
  r : Inport  Port=3
  theta : Inport  Port=4
  Add : Sum  Inputs=+++
  Cos : Trigonometry  Operator=cos
  Integrator : Integrator
  Product : Product  Inputs=3
  Product1 : Product  Inputs=3
  Sin : Trigonometry
  Tan : Trigonometry  Operator=tan
  Tan1 : Trigonometry  Operator=tan
  phi : Outport
  wires:
  p/1 -> Add/1
  Cos/1 -> Product1/1
  Add/1 -> Integrator/1  "phi'"
  Sin/1 -> Product/1
  Tan1/1 -> Product1/2
  Product/1 -> Add/2
  Tan/1 -> Product/2
  Product1/1 -> Add/3
  r/1 -> Product1/3
  theta/1 -> Tan/1, Tan1/1
  q/1 -> Product/3
  Integrator/1 -> Sin/1, Cos/1, phi/1

== system QuadCopterSimulation_CL_Original/	QuadCopter Dynamics/Euler Equations/Subsystem1 ==
  phi : Inport
  r : Inport  Port=2
  q : Inport  Port=3
  Cos : Trigonometry  Operator=cos
  Integrator : Integrator
  Product : Product
  Product1 : Product
  Sin : Trigonometry
  Subtract : Sum  Inputs=+-
  theta : Outport
  wires:
  phi/1 -> Cos/1, Sin/1
  Subtract/1 -> Integrator/1  "theta'"
  Product/1 -> Subtract/2
  Sin/1 -> Product/1
  Integrator/1 -> theta/1
  r/1 -> Product/2
  Cos/1 -> Product1/2
  Product1/1 -> Subtract/1
  q/1 -> Product1/1

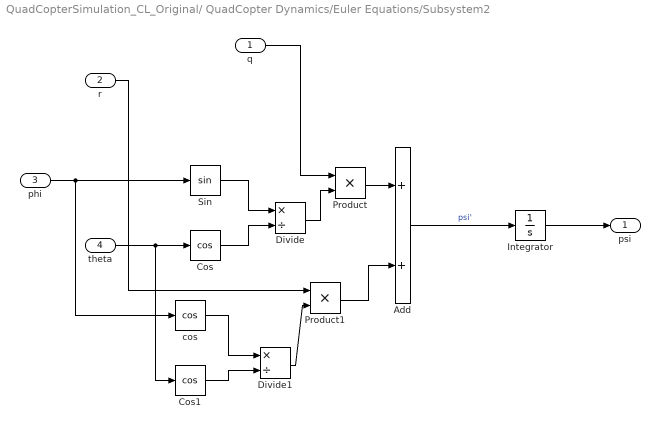
== system QuadCopterSimulation_CL_Original/	QuadCopter Dynamics/Euler Equations/Subsystem2 ==
  q : Inport
  r : Inport  Port=2
  phi : Inport  Port=3
  theta : Inport  Port=4
  Add : Sum
  Cos : Trigonometry  Operator=cos
  Cos1 : Trigonometry  Operator=cos
  Divide : Product  Inputs=*/
  Divide1 : Product  Inputs=*/
  Integrator : Integrator
  Product : Product
  Product1 : Product
  Sin : Trigonometry
  cos : Trigonometry  Operator=cos
  psi : Outport
  wires:
  Divide/1 -> Product/2
  Product1/1 -> Add/2
  Cos/1 -> Divide/2
  Divide1/1 -> Product1/2
  r/1 -> Product1/1
  cos/1 -> Divide1/1
  Cos1/1 -> Divide1/2
  Add/1 -> Integrator/1  "psi'"
  Sin/1 -> Divide/1
  Product/1 -> Add/1
  phi/1 -> cos/1, Sin/1
  Integrator/1 -> psi/1
  theta/1 -> Cos1/1, Cos/1
  q/1 -> Product/1

== system QuadCopterSimulation_CL_Original/	QuadCopter Dynamics/Euler Equations/p_q _r_equations ==
  Tphi : Inport
  Ttheta : Inport  Port=2
  Tpsi : Inport  Port=3
  Subsystem : Subsystem
  Subsystem1 : Subsystem
  Subsystem2 : Subsystem
  p : Outport
  q : Outport  Port=2
  r : Outport  Port=3
  wires:
  Subsystem2/1(r) -> r/1, Subsystem1/3(r), Subsystem/3(r)
  Tpsi/1 -> Subsystem2/1(Tpsi)
  Subsystem1/1(q) -> q/1, Subsystem2/3(q), Subsystem/2(q)
  Subsystem/1(p) -> p/1, Subsystem2/2(p), Subsystem1/2(p)
  Tphi/1 -> Subsystem/1(Tphi)
  Ttheta/1 -> Subsystem1/1(Ttheta)

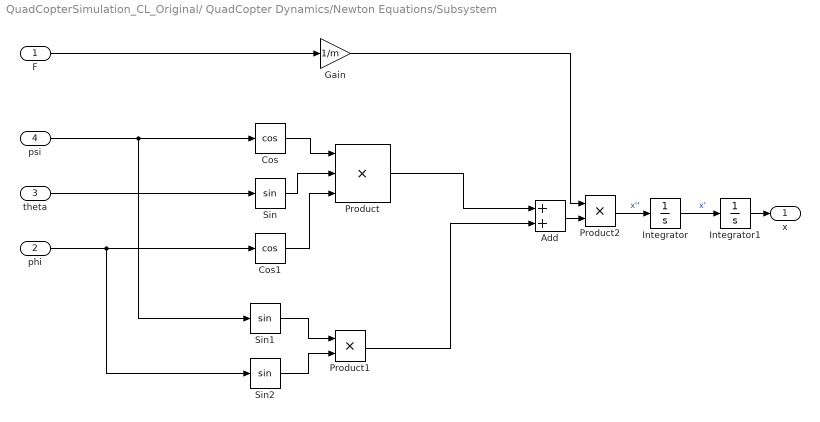
== system QuadCopterSimulation_CL_Original/	QuadCopter Dynamics/Newton Equations/Subsystem ==
  F : Inport
  phi : Inport  Port=2
  theta : Inport  Port=3
  psi : Inport  Port=4
  Add : Sum
  Cos : Trigonometry  Operator=cos
  Cos1 : Trigonometry  Operator=cos
  Gain : Gain  Gain=1/m
  Integrator : Integrator
  Integrator1 : Integrator
  Product : Product  Inputs=3
  Product1 : Product
  Product2 : Product
  Sin : Trigonometry
  Sin1 : Trigonometry
  Sin2 : Trigonometry
  x : Outport
  wires:
  Product1/1 -> Add/2
  Cos1/1 -> Product/3
  psi/1 -> Sin1/1, Cos/1
  Sin1/1 -> Product1/1
  Cos/1 -> Product/1
  phi/1 -> Sin2/1, Cos1/1
  Product/1 -> Add/1
  Sin/1 -> Product/2
  Add/1 -> Product2/2
  Sin2/1 -> Product1/2
  Gain/1 -> Product2/1
  Integrator/1 -> Integrator1/1  "x'"
  Product2/1 -> Integrator/1  "x''"
  F/1 -> Gain/1
  theta/1 -> Sin/1
  Integrator1/1 -> x/1

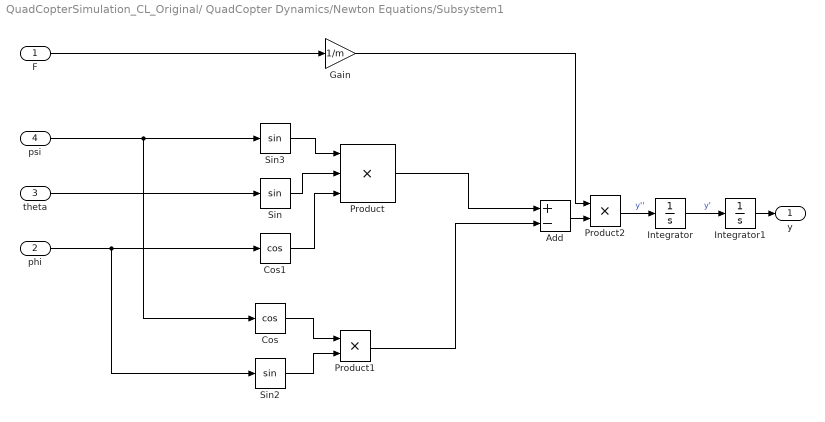
== system QuadCopterSimulation_CL_Original/	QuadCopter Dynamics/Newton Equations/Subsystem1 ==
  F : Inport
  phi : Inport  Port=2
  theta : Inport  Port=3
  psi : Inport  Port=4
  Add : Sum  Inputs=+-
  Cos : Trigonometry  Operator=cos
  Cos1 : Trigonometry  Operator=cos
  Gain : Gain  Gain=1/m
  Integrator : Integrator
  Integrator1 : Integrator
  Product : Product  Inputs=3
  Product1 : Product
  Product2 : Product
  Sin : Trigonometry
  Sin2 : Trigonometry
  Sin3 : Trigonometry
  y : Outport
  wires:
  Integrator1/1 -> y/1
  theta/1 -> Sin/1
  F/1 -> Gain/1
  Product2/1 -> Integrator/1  "y''"
  Integrator/1 -> Integrator1/1  "y'"
  Gain/1 -> Product2/1
  Sin2/1 -> Product1/2
  Add/1 -> Product2/2
  Sin/1 -> Product/2
  Product/1 -> Add/1
  phi/1 -> Cos1/1, Sin2/1
  Sin3/1 -> Product/1
  Cos/1 -> Product1/1
  psi/1 -> Cos/1, Sin3/1
  Cos1/1 -> Product/3
  Product1/1 -> Add/2

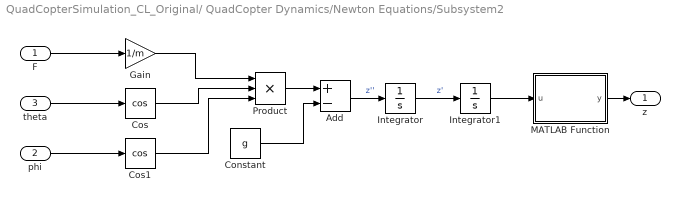
== system QuadCopterSimulation_CL_Original/	QuadCopter Dynamics/Newton Equations/Subsystem2 ==
  F : Inport
  phi : Inport  Port=2
  theta : Inport  Port=3
  Add : Sum  Inputs=+-
  Constant : Constant  Value=g
  Cos : Trigonometry  Operator=cos
  Cos1 : Trigonometry  Operator=cos
  Gain : Gain  Gain=1/m
  Integrator : Integrator
  Integrator1 : Integrator
  MATLAB Function : MATLAB Function  TreatAsAtomicUnit=on
  Product : Product  Inputs=3
  z : Outport
  wires:
  Cos1/1 -> Product/3
  Product/1 -> Add/1
  Integrator/1 -> Integrator1/1  "z'"
  Constant/1 -> Add/2
  theta/1 -> Cos/1
  Gain/1 -> Product/1
  Cos/1 -> Product/2
  Add/1 -> Integrator/1  "z''"
  phi/1 -> Cos1/1
  F/1 -> Gain/1
  Integrator1/1 -> MATLAB Function/1(u)
  MATLAB Function/1(y) -> z/1

== system QuadCopterSimulation_CL_Original/	QuadCopter Dynamics/Euler Equations/p_q _r_equations/Subsystem ==
  Tphi : Inport
  q : Inport  Port=2
  r : Inport  Port=3
  Add : Sum
  Constant : Constant  Value=Iyy-Izz
  Constant1 : Constant  Value=Ixx
  Display : Display
  Divide : Product  Inputs=*/
  Gain : Gain  Gain=1/Ixx
  Integrator : Integrator  AbsoluteTolerance=1e-3
  Product : Product
  Product1 : Product
  p : Outport
  wires:
  Add/1 -> Integrator/1, Display/1  "p'"
  Constant/1 -> Divide/1
  Product/1 -> Add/1
  Gain/1 -> Add/2
  Product1/1 -> Product/2
  Divide/1 -> Product/1
  Constant1/1 -> Divide/2
  Tphi/1 -> Gain/1
  q/1 -> Product1/1
  r/1 -> Product1/2
  Integrator/1 -> p/1

== system QuadCopterSimulation_CL_Original/	QuadCopter Dynamics/Euler Equations/p_q _r_equations/Subsystem1 ==
  Ttheta : Inport
  p : Inport  Port=2
  r : Inport  Port=3
  Add1 : Sum
  Constant2 : Constant  Value=Izz-Ixx
  Constant3 : Constant  Value=Iyy
  Divide1 : Product  Inputs=*/
  Gain1 : Gain  Gain=1/Iyy
  Integrator1 : Integrator
  Product1 : Product
  Product2 : Product
  q : Outport
  wires:
  Integrator1/1 -> q/1
  Add1/1 -> Integrator1/1  "q'"
  Divide1/1 -> Product1/1
  Ttheta/1 -> Gain1/1
  Gain1/1 -> Add1/2
  Constant3/1 -> Divide1/2
  Constant2/1 -> Divide1/1
  Product1/1 -> Add1/1
  Product2/1 -> Product1/2
  p/1 -> Product2/1
  r/1 -> Product2/2

== system QuadCopterSimulation_CL_Original/	QuadCopter Dynamics/Euler Equations/p_q _r_equations/Subsystem2 ==
  Tpsi : Inport
  p : Inport  Port=2
  q : Inport  Port=3
  Add2 : Sum
  Constant4 : Constant  Value=Ixx-Iyy
  Constant5 : Constant  Value=Izz
  Divide2 : Product  Inputs=*/
  Gain2 : Gain  Gain=1/Izz
  Integrator2 : Integrator
  Product1 : Product
  Product2 : Product
  r : Outport
  wires:
  Constant5/1 -> Divide2/2
  Product1/1 -> Product2/2
  Add2/1 -> Integrator2/1  "r'"
  Tpsi/1 -> Gain2/1
  Gain2/1 -> Add2/2
  Divide2/1 -> Product2/1
  Constant4/1 -> Divide2/1
  Product2/1 -> Add2/1
  Integrator2/1 -> r/1
  p/1 -> Product1/1
  q/1 -> Product1/2

== matlab function QuadCopterSimulation_CL_Original/	QuadCopter Dynamics/Newton Equations/Subsystem2/MATLAB Function ==
  data: u input; y output
function y = GndCollision(u)
if u>0
    y=0;
else
y = u;
end
